simulink model "Automatic_Control3"  (R2021a)
settings: Solver=VariableStepAuto  StartTime=0.0  StopTime=13  RelTol=1e-3
values from neighbouring files (symbols this model uses):
  b = 0.006    [Automatic_Control.m]
  b_high = 0.0066    [Automatic_Control.m]
  b_low = 0.0054    [Automatic_Control.m]
  Jm = 0.05    [Automatic_Control.m]
  Jm_high = 0.055    [Automatic_Control.m]
  Jm_low = 0.045    [Automatic_Control.m]
  Ke = 0.05    [Automatic_Control.m]
  Ke_high = 0.055    [Automatic_Control.m]
  Ke_low = 0.045    [Automatic_Control.m]
  Kt = 0.05    [Automatic_Control.m]
  Kt_high = 0.055    [Automatic_Control.m]
  Kt_low = 0.045    [Automatic_Control.m]
  La = 0.01    [Automatic_Control.m]
  La_high = 0.011    [Automatic_Control.m]
  La_low = 0.009    [Automatic_Control.m]
  Ra = 10    [Automatic_Control.m]
  Ra_high = 11.0    (= 11)    [Automatic_Control.m]
  Ra_low = 9.0    (= 9)    [Automatic_Control.m]
undefined symbols (not defined in the file or in its folder): sigbuilder_block
libraries: simulink x2
settings Model: Creator=Rosa  LastModifiedBy=han_jjun_mac
settings SolverCC: AlgebraicLoopSolver=TrustRegion
settings DebuggingCC: SFMachineParentedDataDiag=warning

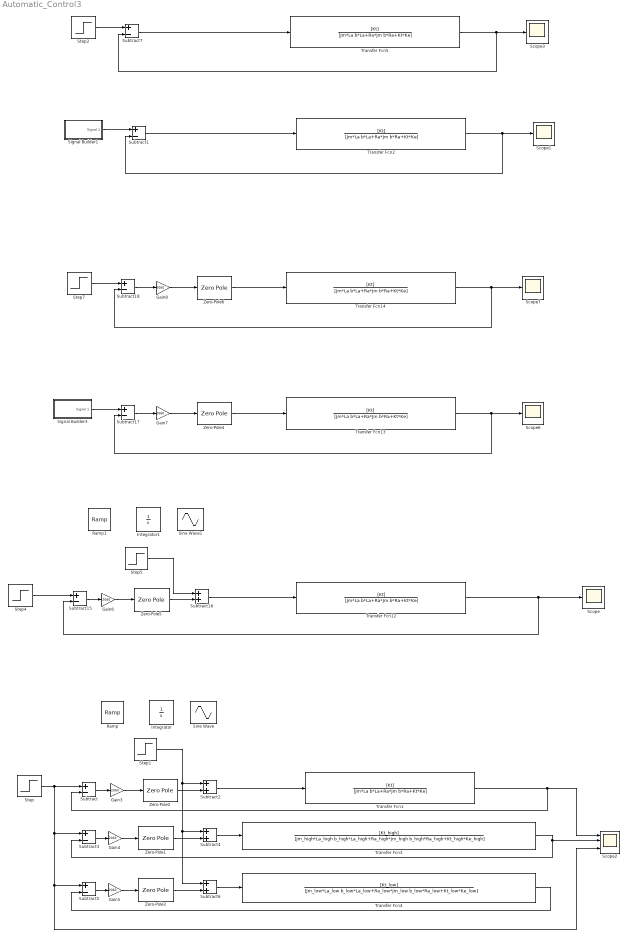
== system Automatic_Control3 ==
  Gain{3..8} (6 alike) : Gain  Gain=2060
  Integrator : Integrator
  Integrator1 : Integrator
  Ramp : simulink/Sources/Ramp  slope=1  start=0  InitialOutput=0
  Ramp1 : simulink/Sources/Ramp  slope=1  start=0  InitialOutput=0
  Scope{,1,3,6..7} (5 alike) : Scope
  Scope2 : Scope  NumInputPorts=4
  Signal Builder1 : Subsystem  Tag=STV Subsys  LoadFcn=sigbuilder_block('load');  StartFcn=sigbuilder_block('start');  StopFcn=sigbuilder_block('stop');  ClipboardFcn=sigbuilder_block('clipboard');  mask(Sigbuilder block){tuvar=[0:10]}
      mask help: Simulink:masks:SigbuilderBlock_MD
      mask init:
      | if ~strcmp(get_param(bdroot(gcbh),'SimulationStatus'),'stopped') tuvar = sigbuilder_block('maskInit'); end
      settings: CopyFcn=sigbuilder_block('copy');  DeleteFcn=sigbuilder_block('delete');  ModelCloseFcn=sigbuilder_block('modelClose');  PreSaveFcn=sigbuilder_block('preSave');  PauseFcn=sigbuilder_block('pause');  ContinueFcn=sigbuilder_block('continue');  NameChangeFcn=sigbuilder_block('namechange');  OpenFcn=sigbuilder_block('open',[278.4 116.4 531 400.2 ]);  CloseFcn=sigbuilder_block('close');
      mask Display: plot(0, 0, 100, 100,[2, 2, 32, 32, 2], [68, 8, 8, 68, 68],[32, 2], [38, 38], [32, 19, 2],[53, 60, 44], [32, 17, 17, 2],[16, 16, 31, 31]);txt = getActiveGroup(gcbh);text(2, 100, txt,'verticalAlignment', 'top');
  Signal Builder3 : Subsystem  Tag=STV Subsys  LoadFcn=sigbuilder_block('load');  StartFcn=sigbuilder_block('start');  StopFcn=sigbuilder_block('stop');  ClipboardFcn=sigbuilder_block('clipboard');  mask(Sigbuilder block){tuvar=[0:10]}
      mask help: Simulink:masks:SigbuilderBlock_MD
      mask init:
      | if ~strcmp(get_param(bdroot(gcbh),'SimulationStatus'),'stopped') tuvar = sigbuilder_block('maskInit'); end
      settings: CopyFcn=sigbuilder_block('copy');  DeleteFcn=sigbuilder_block('delete');  ModelCloseFcn=sigbuilder_block('modelClose');  PreSaveFcn=sigbuilder_block('preSave');  PauseFcn=sigbuilder_block('pause');  ContinueFcn=sigbuilder_block('continue');  NameChangeFcn=sigbuilder_block('namechange');  OpenFcn=sigbuilder_block('open',[278.4 116.4 531 400.2 ]);  CloseFcn=sigbuilder_block('close');
      mask Display: plot(0, 0, 100, 100,[2, 2, 32, 32, 2], [68, 8, 8, 68, 68],[32, 2], [38, 38], [32, 19, 2],[53, 60, 44], [32, 17, 17, 2],[16, 16, 31, 31]);txt = getActiveGroup(gcbh);text(2, 100, txt,'verticalAlignment', 'top');
  Sine Wave : Sin  SampleTime=0
  Sine Wave1 : Sin  SampleTime=0
  Step{,2,4,7} (4 alike) : Step  Time=0  SampleTime=0
  Step1 : Step  SampleTime=0
  Step5 : Step  SampleTime=0
  Subtract{,1,3,5,7,15,17..18} (8 alike) : Sum  Inputs=+-
  Subtract{2,4,6,16} (4 alike) : Sum
  Transfer Fcn{1..2,5,12..14} (6 alike) : TransferFcn  Numerator=[Kt]  Denominator=[Jm*La b*La+Ra*Jm b*Ra+Kt*Ke]
  Transfer Fcn3 : TransferFcn  Numerator=[Kt_high]  Denominator=[Jm_high*La_high b_high*La_high+Ra_high*Jm_high b_high*Ra_high+Kt_high*Ke_high]
  Transfer Fcn4 : TransferFcn  Numerator=[Kt_low]  Denominator=[Jm_low*La_low b_low*La_low+Ra_low*Jm_low b_low*Ra_low+Kt_low*Ke_low]
  Zero-Pole{1..6} (6 alike) : ZeroPole  Zeros=[-1.406]  Poles=[-28.12]
  wires:
  Step/1 -> Scope2/4, Subtract5/1, Subtract3/1, Subtract/1
  Transfer Fcn1/1 -> Scope2/1, Subtract/2
  Subtract2/1 -> Transfer Fcn1/1
  Subtract4/1 -> Transfer Fcn3/1
  Transfer Fcn3/1 -> Scope2/2, Subtract3/2
  Transfer Fcn4/1 -> Subtract5/2
  Gain3/1 -> Zero-Pole2/1
  Subtract6/1 -> Transfer Fcn4/1
  Subtract5/1 -> Gain5/1
  Zero-Pole3/1 -> Subtract6/2
  Step1/1 -> Subtract6/1, Subtract4/1, Subtract2/1
  Subtract/1 -> Gain3/1
  Zero-Pole2/1 -> Subtract2/2
  Subtract3/1 -> Gain4/1
  Gain4/1 -> Zero-Pole1/1
  Zero-Pole1/1 -> Subtract4/2
  Gain5/1 -> Zero-Pole3/1
  Zero-Pole5/1 -> Subtract16/2
  Subtract15/1 -> Gain6/1
  Step5/1 -> Subtract16/1
  Gain6/1 -> Zero-Pole5/1
  Subtract16/1 -> Transfer Fcn12/1
  Transfer Fcn12/1 -> Subtract15/2, Scope/1
  Step4/1 -> Subtract15/1
  Transfer Fcn13/1 -> Scope6/1, Subtract17/2
  Zero-Pole4/1 -> Transfer Fcn13/1
  Subtract17/1 -> Gain7/1
  Signal Builder3/1(Signal 1) -> Subtract17/1
  Gain7/1 -> Zero-Pole4/1
  Gain8/1 -> Zero-Pole6/1
  Step7/1 -> Subtract18/1
  Subtract18/1 -> Gain8/1
  Zero-Pole6/1 -> Transfer Fcn14/1
  Transfer Fcn14/1 -> Subtract18/2, Scope7/1
  Subtract1/1 -> Transfer Fcn2/1
  Transfer Fcn2/1 -> Scope1/1, Subtract1/2
  Signal Builder1/1(Signal 1) -> Subtract1/1
  Step2/1 -> Subtract7/1
  Subtract7/1 -> Transfer Fcn5/1
  Transfer Fcn5/1 -> Subtract7/2, Scope3/1

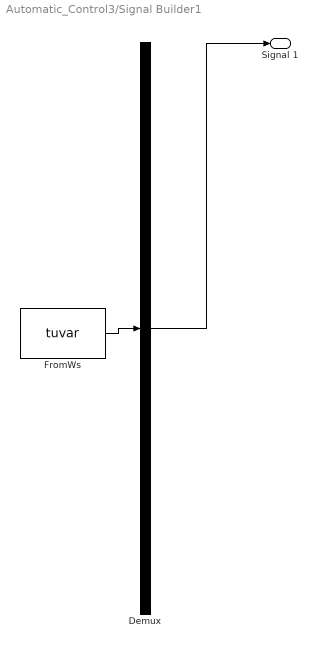
== system Automatic_Control3/Signal Builder1 ==
  Demux : Demux  Tag=STV Demux  Outputs=1
      settings: DisplayOption=none
  FromWs : FromWorkspace  Tag=STV FromWs  VariableName=tuvar
      SigBuilderData=|
      | common.afterFinalStr = 'Extrapolate'
      | common.sampleTime = 0
      | dataSet.timeRange = [0 15]
      | dataSet.name = 'Group 1'
      | sbobj.Groups.Name = 'Group 1'
      | sbobj.Groups.Signals.Name = 'Signal 1'
      | sbobj.Groups.Signals.XData = [0 1 2 10 10 15]
      | sbobj.Groups.Signals.YData = [0 100 100 1 0 0]
      | sbobj.Groups.TimeRange = [0 15]
  Signal 1 : Outport  Tag=STV Outport
  wires:
  FromWs/1 -> Demux/1
  Demux/1 -> Signal 1/1

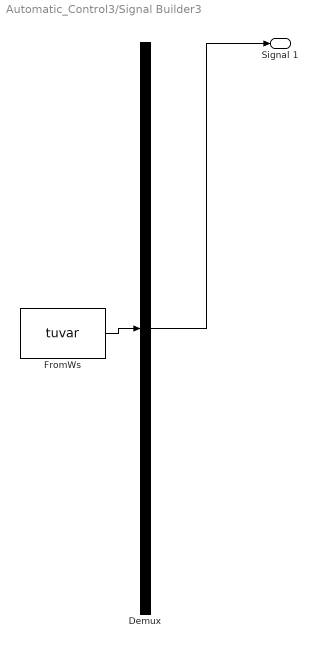
== system Automatic_Control3/Signal Builder3 ==
  Demux : Demux  Tag=STV Demux  Outputs=1
      settings: DisplayOption=none
  FromWs : FromWorkspace  Tag=STV FromWs  VariableName=tuvar
      SigBuilderData=|
      | common.afterFinalStr = 'Extrapolate'
      | common.sampleTime = 0
      | dataSet.timeRange = [0 15]
      | dataSet.name = 'Group 1'
      | sbobj.Groups.Name = 'Group 1'
      | sbobj.Groups.Signals.Name = 'Signal 1'
      | sbobj.Groups.Signals.XData = [0 1 2 10 10 15]
      | sbobj.Groups.Signals.YData = [0 100 100 1 0 0]
      | sbobj.Groups.TimeRange = [0 15]
  Signal 1 : Outport  Tag=STV Outport
  wires:
  FromWs/1 -> Demux/1
  Demux/1 -> Signal 1/1
